simulink model "P42"  (R2015b)
settings: Solver=VariableStepAuto  StartTime=0.0  StopTime=20  RelTol=1e-3
libraries: fl_lib x10, nesl_utility x3
settings Model: Creator=xmax1946  LastModifiedBy=xmax1946

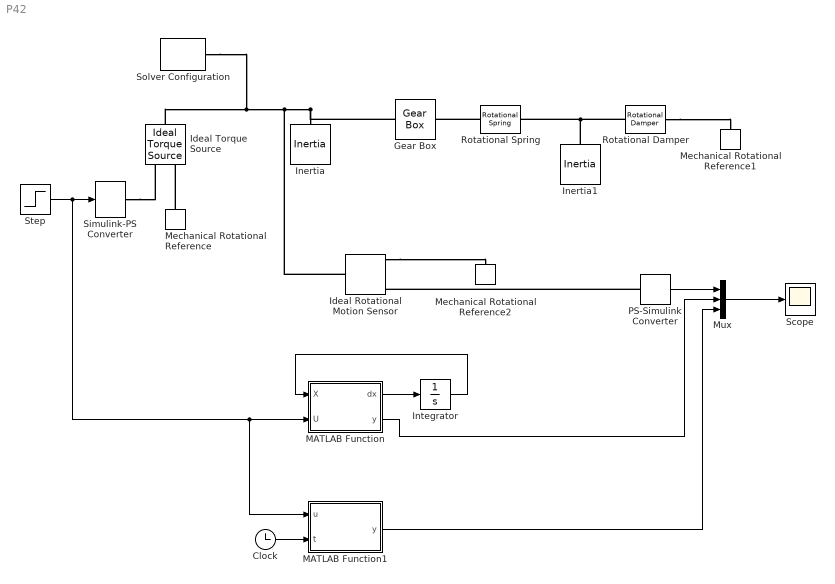
== system P42 ==
  Clock : Clock
  Gear Box : fl_lib/Mechanical/Mechanisms/Gear Box  ratio=100/30  t_in_specify=off  t_in_priority=None  t_in=0 N*m  t_out_specify=off  t_out_priority=None  t_out=0 N*m
  Ideal Rotational Motion Sensor : fl_lib/Mechanical/Mechanical Sensors/Ideal Rotational Motion Sensor  offset=0 rad
  Ideal Torque Source : fl_lib/Mechanical/Mechanical Sources/Ideal Torque Source
  Inertia : fl_lib/Mechanical/Rotational Elements/Inertia  inertia=50 kg*m^2  w_specify=off  w_priority=None  w=0 rad/s  t_specify=off  t_priority=None  t=0 N*m
  Inertia1 : fl_lib/Mechanical/Rotational Elements/Inertia  inertia=100 kg*m^2  w_specify=off  w_priority=None  w=0 rad/s  t_specify=off  t_priority=None  t=0 N*m
  Integrator : Integrator  InitialCondition=[0;0;0;0]
  MATLAB Function : MATLAB Function  TreatAsAtomicUnit=on
  MATLAB Function1 : MATLAB Function  TreatAsAtomicUnit=on
  Mechanical Rotational Reference : fl_lib/Mechanical/Rotational Elements/Mechanical Rotational Reference
  Mechanical Rotational Reference1 : fl_lib/Mechanical/Rotational Elements/Mechanical Rotational Reference
  Mechanical Rotational Reference2 : fl_lib/Mechanical/Rotational Elements/Mechanical Rotational Reference
  Mux : Mux  Inputs=3
  PS-Simulink Converter : nesl_utility/PS-Simulink Converter  PhysicalDomain=network_engine_domain  SubClassName=ps_output  LeftPortType=input  RightPortType=output  PseudoPeriodic=off  Frequencies=[]  Unit=1  AffineConversion=off
  Rotational Damper : fl_lib/Mechanical/Rotational Elements/Rotational Damper  D=100 N*m/(rad/s)  w_specify=off  w_priority=None  w=0 rad/s  t_specify=off  t_priority=None  t=0 N*m
  Rotational Spring : fl_lib/Mechanical/Rotational Elements/Rotational Spring  spr_rate=100 N*m/rad  w_specify=off  w_priority=None  w=0 rad/s  t_specify=off  t_priority=None  t=0 N*m  phi_specify=off  phi_priority=None  phi=0 rad
  Scope : Scope
  Simulink-PS Converter : nesl_utility/Simulink-PS Converter  PhysicalDomain=network_engine_domain  SubClassName=ps_input  LeftPortType=input  RightPortType=output  PseudoPeriodic=off  Frequencies=[]  NoiseDistribution=none  NoiseParameters=[]  Unit=1  AffineConversion=off  InputFiltering=off  SimscapeFilterOrder=1  InputFilterTimeConstant=0.001  UdotUserProvided=1
  Solver Configuration : nesl_utility/Solver Configuration  PhysicalDomain=network_engine_domain  SubClassName=solver  LeftPortType=input  RightPortType=generic  Accelerate=off  Tones=[]  Harmonics=[]  SimulateNoise=off  Profile=off  UseLocalSampling=off  EnableSwitchedLinearOptims=on  FrequencyDomain=off  UseCCode=off  RelTol=0.001  AbsTol=1e-06  MinStep=1e-09  ToWorkspace=off  RevertToSquareIcSolve=off  NumHomotopyIterations=100  PhasorMode=off  PhasorModeNumHarmonics=1  DoDC=off  ResidualTolerance=1e-09  UseLocalSolver=off  LocalSolverChoice=NE_BACKWARD_EULER_ADVANCER  LocalSolverSampleTime=0.001  DoFixedCost=off  MaxNonlinIter=3  MaxModeIter=2  LinearAlgebra=Sparse  DelaysMemoryBudget=1024  AutomaticFiltering=on  FilteringTimeConstant=0.001
  Step : Step  SampleTime=0
  wires:
  Step/1 -> MATLAB Function1/1(u), MATLAB Function/2(U), Simulink-PS Converter/1
  MATLAB Function/1(dx) -> Integrator/1
  Integrator/1 -> MATLAB Function/1(X)
  PS-Simulink Converter/1 -> Mux/1
  Mux/1 -> Scope/1
  MATLAB Function/2(y) -> Mux/2
  Clock/1 -> MATLAB Function1/2(t)
  MATLAB Function1/1(y) -> Mux/3
  connections:
  Ideal Torque Source/LConn1 -- Solver Configuration/RConn1 -- Ideal Rotational Motion Sensor/LConn1 -- Gear Box/LConn1 -- Inertia/LConn1
  Mechanical Rotational Reference/LConn1 -- Ideal Torque Source/RConn2
  Rotational Spring/LConn1 -- Gear Box/RConn1
  Inertia1/LConn1 -- Rotational Damper/LConn1 -- Rotational Spring/RConn1
  Rotational Damper/RConn1 -- Mechanical Rotational Reference1/LConn1
  Simulink-PS Converter/RConn1 -- Ideal Torque Source/RConn1
  Ideal Rotational Motion Sensor/RConn1 -- Mechanical Rotational Reference2/LConn1
  PS-Simulink Converter/LConn1 -- Ideal Rotational Motion Sensor/RConn3

== matlab function P42/MATLAB Function1 ==
  data: u input; y output; t input
function y = fex(u,t)
if(t<1)
y=0;
else
y=(3.9119893329068743761999390280719e-34*u*(0.000000000000000000000000000000041541898769056186572644766503616*exp(0.4131690289707342812519430155926*t + 0.4131690289707342812519430155926)*(9595631571925420296252694710807.0*cos(0.9304772332305556356674428783432*t + 0.9304772332305556356674428783432) + 21609840259293394431880363295177.0*sin(0.9304772332305556356674428783432*t + 0.9304772332305556356674428783432)) - 1.4481704742849844763531537741066) - 7.97083336777119858494997672769e-35*u*(0.000000000000000000000000000000041541898769056186572644766503616*exp(0.4131690289707342812519430155926*t + 0.4131690289707342812519430155926)*(21609840259293394431880363295177.0*cos(0.9304772332305556356674428783432*t + 0.9304772332305556356674428783432) - 9595631571925420296252694710807.0*sin(0.9304772332305556356674428783432*t + 0.9304772332305556356674428783432)) - 0.32754007500974768023252135576676) + 0.11111111111111111111111111111111*t*u - 5.3950598246104543293681451168914e-34*u*(exp(0.17366194205853143749611396881481*t) - 1.0) - 0.73197075004154340919123607422679*u*exp(-0.17366194205853143749611396881481*t)*(exp(0.17366194205853143749611396881481*t) - 1.0) - 7.0430016448812857378970567278463e-34*u*exp(-0.17366194205853143749611396881481*t)*(0.000000000000000000000000000000041541898769056186572644766503616*exp(0.4131690289707342812519430155926*t + 0.4131690289707342812519430155926)*(9595631571925420296252694710807.0*cos(0.9304772332305556356674428783432*t + 0.9304772332305556356674428783432) + 21609840259293394431880363295177.0*sin(0.9304772332305556356674428783432*t + 0.9304772332305556356674428783432)) - 1.4481704742849844763531537741066) + 1.016800730062916766878768429678e-34*u*exp(-0.17366194205853143749611396881481*t)*(0.000000000000000000000000000000041541898769056186572644766503616*exp(0.4131690289707342812519430155926*t + 0.4131690289707342812519430155926)*(21609840259293394431880363295177.0*cos(0.9304772332305556356674428783432*t + 0.9304772332305556356674428783432) - 9595631571925420296252694710807.0*sin(0.9304772332305556356674428783432*t + 0.9304772332305556356674428783432)) - 0.32754007500974768023252135576676) - 6.8004402693071875156074314833537e-34*u*exp(-0.4131690289707342812519430155926*t)*cos(0.9304772332305556356674428783432*t)*(exp(0.17366194205853143749611396881481*t) - 1.0) + 6.4132871058259832919897725523823e-34*u*exp(-0.4131690289707342812519430155926*t)*sin(0.9304772332305556356674428783432*t)*(exp(0.17366194205853143749611396881481*t) - 1.0) - 0.0042602670915698259856906183039547*u*exp(-0.4131690289707342812519430155926*t)*cos(0.9304772332305556356674428783432*t)*(0.000000000000000000000000000000041541898769056186572644766503616*exp(0.4131690289707342812519430155926*t + 0.4131690289707342812519430155926)*(9595631571925420296252694710807.0*cos(0.9304772332305556356674428783432*t + 0.9304772332305556356674428783432) + 21609840259293394431880363295177.0*sin(0.9304772332305556356674428783432*t + 0.9304772332305556356674428783432)) - 1.4481704742849844763531537741066) - 0.00033975629829118624182583709176744*u*exp(-0.4131690289707342812519430155926*t)*sin(0.9304772332305556356674428783432*t)*(0.000000000000000000000000000000041541898769056186572644766503616*exp(0.4131690289707342812519430155926*t + 0.4131690289707342812519430155926)*(9595631571925420296252694710807.0*cos(0.9304772332305556356674428783432*t + 0.9304772332305556356674428783432) + 21609840259293394431880363295177.0*sin(0.9304772332305556356674428783432*t + 0.9304772332305556356674428783432)) - 1.4481704742849844763531537741066) - 0.00033975629829118624182583709176736*u*exp(-0.4131690289707342812519430155926*t)*cos(0.9304772332305556356674428783432*t)*(0.000000000000000000000000000000041541898769056186572644766503616*exp(0.4131690289707342812519430155926*t + 0.4131690289707342812519430155926)*(21609840259293394431880363295177.0*cos(0.9304772332305556356674428783432*t + 0.9304772332305556356674428783432) - 9595631571925420296252694710807.0*sin(0.9304772332305556356674428783432*t + 0.9304772332305556356674428783432)) - 0.32754007500974768023252135576676) + 0.0042602670915698259856906183039548*u*exp(-0.4131690289707342812519430155926*t)*sin(0.9304772332305556356674428783432*t)*(0.000000000000000000000000000000041541898769056186572644766503616*exp(0.4131690289707342812519430155926*t + 0.4131690289707342812519430155926)*(21609840259293394431880363295177.0*cos(0.9304772332305556356674428783432*t + 0.9304772332305556356674428783432) - 9595631571925420296252694710807.0*sin(0.9304772332305556356674428783432*t + 0.9304772332305556356674428783432)) - 0.32754007500974768023252135576676) + 0.0098565651311550631000910431464088);    
end

== matlab function P42/MATLAB Function ==
  data: dx output; X input; y output; U input
function [dx,y] = fss(X,U)
A=[0,1,0,0
   -9/50,0,9/50,0
   0,0,0,1
   1,0,-1,-1];
B=[0;1/50;0;0];
C=[1,0,0,0];
u=U;
dx=A*X+B*u;
y=C*X;
